simulink library "Lib_PFSys_DCDCConv_TMATS"  (R2017a)
settings: Solver=ode45  StartTime=0.0  StopTime=10.0  RelTol=1e-3  EnableMultiTasking=on
libraries: Lib_PF_BusLoadDC_TMATS x1, Lib_PF_ActiveConvEffDC2DC_TMATS x1
Description:
  | Thomas Modules
settings Model: Creator=jwchapm2  LastModifiedBy=glthoma1
settings DataIOCC: LimitDataPoints=on  SaveFormat=Array
settings OptimizationCC: ExpressionDepthLimit=2147483647  LifeSpan=inf
settings DebuggingCC: UnderspecifiedInitializationDetection=Classic  MergeDetectMultiDrivingBlocksExec=none  SolverPrmCheckMsg=warning  StateNameClashWarn=warning  SFUnexpectedBacktrackingDiag=warning  SFNoUnconditionalDefaultTransitionDiag=warning  SFExecutionAtInitializationDiag=none
settings HardwareCC: ProdBitPerPointer=32  ProdBitPerSizeT=32  ProdBitPerPtrDiffT=32  ProdLargestAtomicFloat=None  ProdIntDivRoundTo=Undefined  ProdEndianess=Unspecified  ProdWordSize=32  ProdHWDeviceType=32-bit Generic
settings ModelReferenceCC: PropagateSignalLabelsOutOfModel=off
settings GRTTargetCC: TargetLangStandard=C89/C90 (ANSI)  GeneratePreprocessorConditionals=Disable all
settings ConfigComp: CovMetricSettings=dw  CovHtmlReporting=on  CovSaveCumulativeToWorkspaceVar=on  CovSaveSingleToWorkspaceVar=on  CovExternalEMLEnable=off

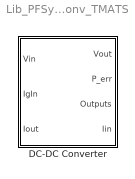
== system Lib_PFSys_DCDCConv_TMATS ==
  DC-DC Converter : Subsystem  mask(DC-DC Converter){X_C_VoltageVec_M=[0.0 0.1 1.0], Y_C_CurrentVec_M=[0.0 0.1 1.0], T_C_EffArray_M=[0.5 0.5 0.5; 0.5 1.0 1.0; 0.5 1.0 1.0], Vout_M=10000, Pdis_M=1}
      mask prompts: X_C_VoltageVec_M "X_C_VoltageVec_M - Efficiency Table Voltage Vector (X-axis)(nx1), V"; Y_C_CurrentVec_M "Y_C_CurrentVec_M - Efficiency Table Current Vector (Y-axis)(mx1), A"; T_C_EffArray_M "T_C_EffArray_M - Efficiency Table Values (Eff = f(i, V)(nxm), Frac"; Vout_M "Vout_M - Output Voltage, V"; Pdis_M "Pdis_M - Constant Power Leaked/Dissipated, W"
      mask help:
      | This block represents a generic DC-DC converter controlled to produce a
      | constant output voltage (either a buck, boost, buck-boost, Cuk, etc.).
      | The converter's efficiency is defined via a lookup table that is a function
      | of input voltage and current. The input current is solved for, such that
      | the power in equals the power out.

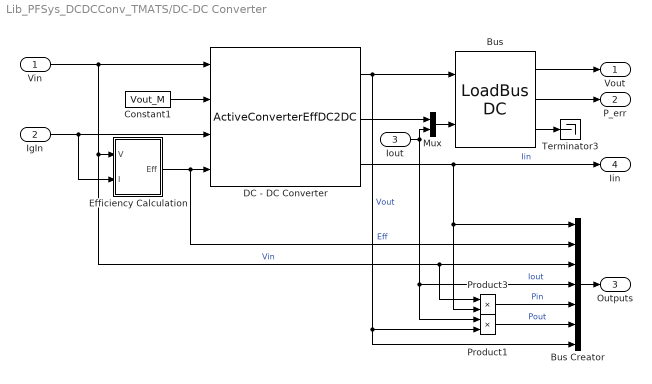
== system Lib_PFSys_DCDCConv_TMATS/DC-DC Converter ==
  Vin : Inport
  IgIn : Inport  Port=2
  Iout : Inport  Port=3
  Bus : Lib_PF_BusLoadDC_TMATS/LoadBus DC  PeInEN_M=off  P_M=-Pdis_M  BlkNm_M=double(gcb)
  Bus Creator : BusCreator  Inputs=7
  Constant1 : Constant  Value=Vout_M
  DC - DC Converter : Lib_PF_ActiveConvEffDC2DC_TMATS/ActiveConverterEffDC2DC  EffInEN_M=on  Eff_M=98  BlkNm_M=double(gcb)
  Efficiency Calculation : Subsystem
  Mux : Mux  Inputs=2
  Product1 : Product
  Product3 : Product
  Terminator3 : Terminator
  Vout : Outport
  P_err : Outport  Port=2
  Outputs : Outport  Port=3
  Iin : Outport  Port=4
  wires:
  Bus/1 -> Vout/1
  Product1/1 -> Bus Creator/6  "Pout"
  Product3/1 -> Bus Creator/5  "Pin"
  Bus Creator/1 -> Outputs/1
  Efficiency Calculation/1(Eff) -> Bus Creator/2, DC - DC Converter/4  "Eff"
  Iout/1 -> Bus Creator/4, Product1/1, Mux/2  "Iout"
  Vin/1 -> DC - DC Converter/1, Bus Creator/3, Product3/1, Efficiency Calculation/1(V)  "Vin"
  IgIn/1 -> DC - DC Converter/3, Efficiency Calculation/2(I)
  Constant1/1 -> DC - DC Converter/2
  DC - DC Converter/2 -> Mux/1
  DC - DC Converter/3 -> Product3/2, Bus Creator/1, Iin/1  "Iin"
  DC - DC Converter/1 -> Bus/1, Bus Creator/7, Product1/2  "Vout"
  Mux/1 -> Bus/2
  Bus/3 -> Terminator3/1
  Bus/2 -> P_err/1

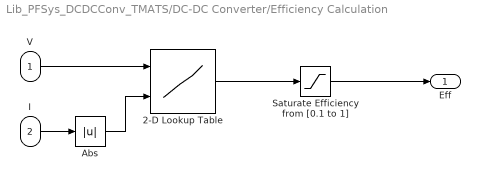
== system Lib_PFSys_DCDCConv_TMATS/DC-DC Converter/Efficiency Calculation ==
  V : Inport
  I : Inport  Port=2
  2-D Lookup Table : Lookup_n-D  BreakpointsForDimension1=X_C_VoltageVec_M  BreakpointsForDimension2=Y_C_CurrentVec_M  Table=T_C_EffArray_M  ExtrapMethod=Clip  InternalRulePriority=Speed  RndMeth=Simplest  InputSameDT=on
  Abs : Abs
  Saturate Efficiency from [0.1 to 1] : Saturate  UpperLimit=1  LowerLimit=0.1
  Eff : Outport
  wires:
  Saturate Efficiency from [0.1 to 1]/1 -> Eff/1
  V/1 -> 2-D Lookup Table/1
  Abs/1 -> 2-D Lookup Table/2
  I/1 -> Abs/1
  2-D Lookup Table/1 -> Saturate Efficiency from [0.1 to 1]/1
